simulink model "F16ASYM_Controlled_AoA"  (R2012b)
settings: Solver=ode3  SolverMode=SingleTasking  StartTime=0.0  StopTime=inf  FixedStep=T_sim  RelTol=1e-3
InitFcn:
  | load('NN_c_weights_Last_stable.mat')
values from neighbouring files (symbols this model uses):
  K_b_AoA = params(3)    [Cost_function.m]
  K_b_q = params(4)    [Cost_function.m]
  learning = 20    [Scheduling_desing.m]
  Model_used_flag = 1    [Scheduling_desing.m]
  reg_param = 0.5    [Scheduling_desing.m]
  T_sim = 0.02    [Scheduling_desing.m]
  tau_AoA = params(1)    [Cost_function.m]
  tau_q = params(2)    [Cost_function.m]
  Theta_1_roll_last = [0.00183613313267 0.00115998993235 0.0006676025148 0.00194921904952 0.00134963559861 0.00034352059664 0.000447169388141 0.00146749660935 0.00110199952389 7.77922383894e-05 0.00109492833348 0.00192687590535 ... (360 elements, 30x12)]    [NN_i_weights_LAST_STABLE.mat]
  Theta_2_roll_last = [0.000469743069697 0.000355923851088 0.00180035760697 0.00191855117771 0.00118851504447 0.0013331642065 0.0013164316578 0.000643981263341 0.00176817665434 0.000113802099363 0.000426534542462 0.00113815782354 ... (620 elements, 20x31)]    [NN_i_weights_LAST_STABLE.mat]
  Theta_3_roll_last = [9.62071520568e-05 -0.000389870886846 2.08260845013e-05 0.000140787743673 -0.000917525755397 -0.0014324207578 -0.00154701573815 -0.00131544476264 -0.00101205584381 5.06515794689e-05 -0.00111443483676 -0.00143957416141 ... (21 elements, 1x21)]    [NN_i_weights_LAST_STABLE.mat]
  V_long_lastA_w_z = [0.352826086601 -0.253633004548 -0.642535042878 0.237749930435 -0.618390629538 0.858074761295 0.268211230628 -0.448715080196 -0.0406384631192 0.401147605577 0.60598427709 0.0500551915851 ... (300 elements, 30x10)]    [NN_i_weights_LAST_STABLE.mat]
  V_long_lastAoA = [0.0774300162379 0.0911421319631 0.0352371192557 0.0542170286952 0.0651171200844 0.0177112012707 0.0982957728448 0.000259994642558 0.0194724569123 0.0466321328252 0.0556687953852 0.0252668067142 ... (300 elements, 30x10)]    [NN_i_weights_LAST_STABLE.mat]
  V_roll_last = [0.0540918675943 0.0557493347212 0.0839792276608 0.0460576391794 0.0671229058124 0.100220403067 0.0722493281881 0.0648875457457 0.00447599349201 0.0607299103823 0.0488037966361 0.0176785979393 ... (360 elements, 30x12)]    [NN_i_weights_LAST_STABLE.mat]
  V_yaw_last = [0.0965149149679 0.00833616709545 0.0365734360076 0.0523944217566 0.00790252078455 0.0700053845887 0.0345164868709 0.0111568465295 0.094060639546 0.0205483560006 0.000798047494256 0.0862769385758 ... (360 elements, 30x12)]    [NN_i_weights_LAST_STABLE.mat]
  velocity = M_eval_sche(I,J)*a    [Scheduling_desing.m]
  W_long_lastA_w_z = [-0.0522913429974 0.00385484301394 -0.00465489482472 -0.0139416219936 0.00295196421483 -0.013027768541 0.00585545058915 0.00278802233571 -0.00906272782329 -0.000396112031465 0.00405849743321 0.00509668457818 ... (31 elements, 1x31)]    [NN_i_weights_LAST_STABLE.mat]
  W_long_lastAoA = [-0.0192589013922 0.00873109909713 0.00432649597332 0.0420946902441 0.0293366820194 0.0351497798191 0.0234952374236 0.0360841187718 0.0112233388211 0.030147202199 0.0369533138617 0.00218839076415 ... (31 elements, 1x31)]    [NN_i_weights_LAST_STABLE.mat]
  W_roll_last = [-0.0006515532842 0.000535485585715 0.000550946920743 0.000806030945453 0.00045976209382 0.00065557954304 0.000945902185602 0.00070191398535 0.000635215543728 4.66501377412e-05 0.000597079583757 0.000485790566765 ... (31 elements, 1x31)]    [NN_i_weights_LAST_STABLE.mat]
  W_yaw_last = [-4.34263633305e-05 8.83823048922e-05 1.65575463724e-05 3.60293102233e-05 5.19752447623e-05 7.06399280852e-06 7.02425975821e-05 3.62680255076e-05 1.29996379937e-05 8.05072914397e-05 2.39941870661e-05 2.52427840574e-06 ... (31 elements, 1x31)]    [NN_i_weights_LAST_STABLE.mat]
undefined symbols (not defined in the file or in its folder): a1, alpha_map_eval, B, beta_map_eval, C_L_0, DiscIntNeverNeededParam, fi_flag_Simulink, G_eval, H_sq, H_sq_autotrim, k_B, m_B, M_sq, M_sq_autotrim, sigbuilder_block, Stall_curve, trim_control, trim_state, trim_throttle, V_Comp_A_w_z_last, V_Comp_last, V_roll_lastMOD, W_Comp_A_w_z_last, W_Comp_last, W_roll_lastMOD
libraries: Adaptive_FaultTolerantControl x43, dspsigops x29, F16_Actuator_Library x14, simulink x8, aerolibatmos2 x7, dsparch4 x6, simulink_extras x5, aerolibtransform2 x5, qcatlib x4, dspmtrx3 x3, dspvision x2, dspsnks4 x2
(part 1 of 11)
settings Model: MAModelExclusionFile=C:\Users\David\Documents\Estudios y formación academica\Cranfield\Thesis F16\Work\Solutions\7dof Base\F16ASYM_Controlled_exclusions.xml  Creator=David  LastModifiedBy=David
settings SolverCC: AutoInsertRateTranBlk=on
settings DataIOCC: SaveOutput=off  SignalLogging=off  DSMLogging=off  SaveTime=off
settings OptimizationCC: BlockReduction=off  InlineParams=on  InlineInvariantSignals=on  EnableMemcpy=off  StateBitsets=on  DataBitsets=on  UseTempVars=on  ZeroExternalMemoryAtStartup=off  ZeroInternalMemoryAtStartup=off  NoFixptDivByZeroProtection=on  EfficientMapNaN2IntZero=off  OptimizeModelRefInitCode=on  LifeSpan=1
settings HardwareCC: ProdIntDivRoundTo=Floor  ProdEndianess=LittleEndian  ProdHWDeviceType=Generic->Custom
settings RTWCC: SystemTargetFile=ert.tlc  TLCOptions=-p0  GenCodeOnly=on  TemplateMakefile=ert_default_tmf  Description=Embedded Coder  GenerateReport=on  RTWVerbose=off  ProcessScript=ert_make_rtw_hook  IncludeHyperlinkInReport=on  LaunchReport=on
settings CodeAppCC: ForceParamTrailComments=on  IgnoreCustomStorageClasses=off  SimulinkDataObjDesc=on  CustomSymbolStrGlobalVar=rt$N$M  CustomSymbolStrType=$N$M  CustomSymbolStrFcn=$N$M$F  CustomSymbolStrMacro=$N$M  InsertBlockDesc=on
settings ERTTargetCC: CodeReplacementLibrary=ISO_C  MultiwordLength=2048  GenerateSampleERTMain=on  IncludeMdlTerminateFcn=off  SuppressErrorStatus=on  SupportAbsoluteTime=off  SupportNonFinite=off  SupportComplex=off  PurelyIntegerCode=on  InlinedParameterPlacement=NonHierarchical  RootIOFormat=Structure reference  ERTCustomFileTemplate=example_file_process.tlc  ConvertIfToSwitch=off  SuppressUnreachableDefaultCases=off

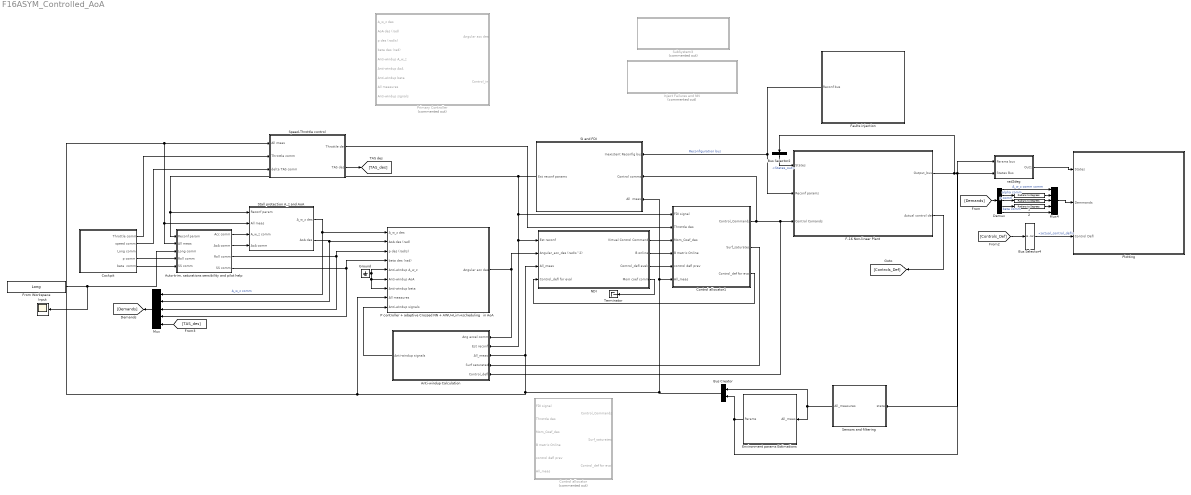
== system F16ASYM_Controlled_AoA ==
  "  " : simulink_extras/Transformations/Radians to Degrees
  "  1" : simulink_extras/Transformations/Radians to Degrees
  "  2" : simulink_extras/Transformations/Radians to Degrees
  Anti-windup Calculation : Subsystem  Variant=on  OverrideUsingVariant=Reconfigurable
  "Auto-trim, saturations sensibility and pilot help" : Subsystem
  Bus Creator : BusCreator  Inputs=2
  Bus Selector2 : BusSelector  OutputSignals=States_out
  Bus Selector4 : BusSelector  OutputSignals=actual_control_defl
  Cockpit : Subsystem
      mask Display:
      | image(imread('Cockpit2.jpg'))
      | 
      | port_label('output', 1, 'Throttle comm')
      | port_label('output', 2, 'Speed comm')
      | port_label('output', 3, 'Long comm')
      | port_label('output', 4, 'p comm')
      | port_label('output', 5, 'beta comm')
  Control allocator : Subsystem  Commented=on  Variant=on  OverrideUsingVariant=Control Allocator: NO RECONFIG
  Control allocator1 : Subsystem  Variant=on  OverrideUsingVariant=Control Allocator: RECONFIG
  Demux : Demux  Outputs=5
  Environment params Estimations : Subsystem
  F-16 Non-linear Plant : Subsystem  Variant=on  OverrideUsingVariant=Reconfigurable
      mask Display:
      | image(imread('f16.jpg'))
      | 
      | port_label('output', 1, 'Out_bus')
      | port_label('output', 2, 'Actual Control deflec')
      | 
      | port_label('input', 1, 'State_feedback')
      | port_label('input', 2, 'Reconf_params')
      | port_label('input', 3, 'Control_Commands')
      | 
      | % Variant dealing
      | ActiveVar = get_param(gcb,'activevariant');
      | 
      | 
      | disp(['{\bf\fontsize{16}',ActiveVar,'}'], 'texmode','on');
  Faults injection : Subsystem
      settings: OpenFcn=Control_GUI
      mask Display: disp(['{\bf \fontsize{16}',sprintf('Faults \n and\n  deviations\n  injection'),'}'], 'texmode','on');
  From Workspace : FromWorkspace  VariableName=Long  SampleTime=T_sim
  Ground : Ground
  Inject Failures and NN : Subsystem  Commented=on
      settings: OpenFcn=Control_GUI
      mask Display: disp('Inject Failures & NN management GUI')
  Input : Scope
      settings: YMin=-20  YMax=35  SaveName=ScopeData29
  Mux : Mux  Inputs=[1 1 1 1 1]
  Mux4 : Mux  Inputs=5
  NDI : Subsystem  Variant=on  OverrideUsingVariant=NDI: RECONFIG
  P controller + adaptive Crossed NN + AWU+Lim+scheduling   in AoA : Subsystem  VariantObject=Adaptive Controller Crossed+AWU+Lim
  Plotting : Subsystem
      mask Display:
      | disp('{\bf\fontsize{20} Plotting}', 'texmode','on');
      | % port_label('input', 1, 'States')
      | % port_label('input', 2, 'Demans')
  Primary Controller : Subsystem  Commented=on  Variant=on  OverrideUsingVariant=Adaptive Controller Crossed+AWU+Lim+hand-over
  SI and FDI : Subsystem  Variant=on  OverrideUsingVariant=Realistic
      mask Display:
      | % Variant dealing
      | ActiveVar = get_param(gcb,'activevariant');
      | 
      | 
      | 
      | disp(['{\bf \fontsize{14}',sprintf('SI \n&\nFDI\n\n '),ActiveVar,'}'], 'texmode','on');
  Sensors and filtering : Subsystem
  Speed-Throttle control : Subsystem
  Stall protection A_z and AoA : Subsystem  Variant=on  OverrideUsingVariant=Using AoA
  SubSystem3 : Subsystem  Commented=on
      settings: OpenFcn=FE_plot
      mask Display:
      | % image(imread('FE.png'))
      | 
      | disp('Flight Envelope position');
  Terminator : Terminator
  rad2deg : Subsystem
  wires:
  Sensors and filtering/1(All_measures) -> Environment params Estimations/1(All_meas), Bus Creator/1
  Control allocator1/2(Surf_saturated) -> Anti-windup Calculation/4(Surf saturated)
  NDI/1(Virtual Control Commands) -> Control allocator1/3(Mom_Coef_des)
  Ground/1 -> P controller + adaptive Crossed NN + AWU+Lim+scheduling   in AoA/7(Anti-windup beta), P controller + adaptive Crossed NN + AWU+Lim+scheduling   in AoA/6(Anti-windup AoA), P controller + adaptive Crossed NN + AWU+Lim+scheduling   in AoA/5(Anti-windup A_w_z)
  Bus Selector2/1 -> F-16 Non-linear Plant/1(States)  "<States_out>"
  NDI/2(B online) -> Control allocator1/4(B matrix Online)
  F-16 Non-linear Plant/2(Actual control def) -> [Controls_Def]
  P controller + adaptive Crossed NN + AWU+Lim+scheduling   in AoA/1(Angular acc des) -> NDI/2(Angular_acc_des (rad/s^2)), Anti-windup Calculation/1(Ang accel comm)
  NDI/3(Control_defl evald) -> Control allocator1/5(control defl prev)
  Control allocator1/3(Control_def for eval) -> NDI/4(Control_defl for eval)
  Faults injection/1(Reconf bus) -> F-16 Non-linear Plant/2(Reconf params), SI and FDI/1(Inexistent Reconfig bus)  "Reconfiguration bus"
  Control allocator1/1(Control_Commands) -> SI and FDI/2(Control comms), F-16 Non-linear Plant/3(Control Comands), Anti-windup Calculation/5(Control_defl)
  Bus Creator/1 -> Control allocator1/6(All_meas), SI and FDI/3(All  meas), P controller + adaptive Crossed NN + AWU+Lim+scheduling   in AoA/8(All measures), "Auto-trim, saturations sensibility and pilot help"/2(All meas), Stall protection A_z and AoA/2(All meas), Speed-Throttle control/1(All meas), NDI/3(All_meas), Anti-windup Calculation/3(All_meas)
  "Auto-trim, saturations sensibility and pilot help"/1(Acc comm) -> Stall protection A_z and AoA/3(A_w_z comm)
  Anti-windup Calculation/1(Anti-windup signals) -> P controller + adaptive Crossed NN + AWU+Lim+scheduling   in AoA/9(Anti-windup signals)
  Stall protection A_z and AoA/1(A_w_z des) -> Mux/1, P controller + adaptive Crossed NN + AWU+Lim+scheduling   in AoA/1(A_w_z des)  "A_w_z comm"
  "Auto-trim, saturations sensibility and pilot help"/4("SS comm ") -> P controller + adaptive Crossed NN + AWU+Lim+scheduling   in AoA/4(beta des (rad)), Mux/4
  "Auto-trim, saturations sensibility and pilot help"/3("Roll comm ") -> P controller + adaptive Crossed NN + AWU+Lim+scheduling   in AoA/3(p des (rad/s)), Mux/3
  SI and FDI/1(Est reconf params) -> "Auto-trim, saturations sensibility and pilot help"/1(Reconf param), Stall protection A_z and AoA/1(Reconf param), Control allocator1/1(FDI signal), Anti-windup Calculation/2(Est reconf), NDI/1(Est reconf)
  Cockpit/4(p comm) -> "Auto-trim, saturations sensibility and pilot help"/4(Roll comm)
  Cockpit/5(beta  comm) -> "Auto-trim, saturations sensibility and pilot help"/5(SS comm)
  "Auto-trim, saturations sensibility and pilot help"/2(AoA comm) -> Stall protection A_z and AoA/4(AoA comm)
  Cockpit/1(Throttle comm) -> Speed-Throttle control/2(Throttle comm)
  Cockpit/2(speed comm) -> Speed-Throttle control/3(delta TAS comm)
  Speed-Throttle control/1(Throttle des) -> Control allocator1/2(Throttle des)
  Mux/1 -> [Demands]
  Speed-Throttle control/2(TAS des) -> [TAS_des]
  [TAS_des] -> Mux/5
  Stall protection A_z and AoA/2(AoA des) -> Mux/2, P controller + adaptive Crossed NN + AWU+Lim+scheduling   in AoA/2(AoA des (rad))
  From Workspace/1 -> "Auto-trim, saturations sensibility and pilot help"/3(Long comm), Input/1
  NDI/4(Mom coef comm) -> Terminator/1
  rad2deg/1(Out1) -> Plotting/1(States)
  F-16 Non-linear Plant/1(Output_bus) -> rad2deg/2(States Bus), Sensors and filtering/1(state), Bus Selector2/1
  [Demands] -> Demux/1
  Environment params Estimations/1(Params) -> Bus Creator/2, rad2deg/1(Params bus)
  Demux/3 -> "  1"/1  "p comm"
  Demux/4 -> "  2"/1  "beta comm"
  Demux/2 -> "  "/1  "alpha comm"
  Mux4/1 -> Plotting/2(Demmands)
  Demux/1 -> Mux4/1  "A_w_z comm comm"
  "  "/1 -> Mux4/2
  "  1"/1 -> Mux4/3
  "  2"/1 -> Mux4/4
  [Controls_Def] -> Bus Selector4/1
  Bus Selector4/1 -> Plotting/3(Control Defl)  "<actual_control_defl>"
  Demux/5 -> Mux4/5

== system F16ASYM_Controlled_AoA/Anti-windup Calculation ==
  Ang accel comm : Inport
  Est reconf : Inport  Port=2
  All_meas : Inport  Port=3
  Surf saturated : Inport  Port=4
  Control_defl : Inport  Port=5
  Anti-windup: NO reconfigurable : Subsystem  VariantObject=No reconfigurable
  Anti-windup: Reconfigurable : Subsystem  VariantObject=Reconfigurable
  Anti-windup signals : Outport

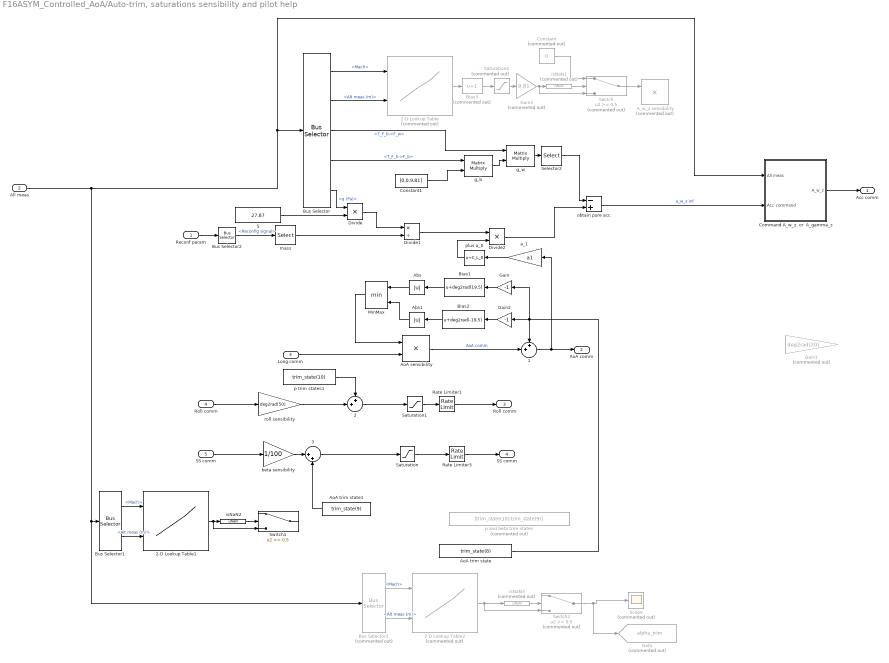
== system F16ASYM_Controlled_AoA/Auto-trim, saturations sensibility and pilot help ==
  Reconf param : Inport
  All meas : Inport  Port=2
  Long comm : Inport  Port=3
  Roll comm : Inport  Port=4
  SS comm : Inport  Port=5
  " 1" : Sum  Inputs=++|
  " 2" : Sum  Inputs=++|
  " 3" : Sum  Inputs=|++
  2-D Lookup Table : Lookup_n-D  Commented=on  BreakpointsForDimension1=M_sq  BreakpointsForDimension2=H_sq  Table=G_eval  RemoveProtectionInput=on  SampleTime=5*T_sim  RndMeth=Simplest  InputSameDT=on
  2-D Lookup Table1 : Lookup_n-D  BreakpointsForDimension1=M_sq_autotrim  BreakpointsForDimension2=H_sq_autotrim  Table=beta_map_eval  RemoveProtectionInput=on  SampleTime=5*T_sim  RndMeth=Simplest  InputSameDT=on
  2-D Lookup Table2 : Lookup_n-D  Commented=on  BreakpointsForDimension1=M_sq_autotrim  BreakpointsForDimension2=H_sq_autotrim  Table=alpha_map_eval  RemoveProtectionInput=on  SampleTime=5*T_sim  RndMeth=Simplest  InputSameDT=on
  A_w_z sensibility : Product  Commented=on  Inputs=**
  Abs : Abs
  Abs1 : Abs
  AoA sensibility : Product  Inputs=**
  AoA trim state : Constant  Value=trim_state(8)
  AoA trim state1 : Constant  Value=trim_state(9)
  Bias1 : Bias  Bias=deg2rad(19.5)
  Bias2 : Bias  Bias=deg2rad(-19.5)
  Bias3 : Bias  Commented=on  Bias=1
  Bus Selector : BusSelector  OutputSignals=signal2.Mach,signal1.Alt meas (m),signal2.T_F_b->F_w,signal2.T_F_h->F_b,signal2.q (Pa)
  Bus Selector1 : BusSelector  OutputSignals=signal2.Mach,signal1.Alt meas (m)
  Bus Selector2 : BusSelector  OutputSignals=Reconfig signal
  Bus Selector3 : BusSelector  Commented=on  OutputSignals=signal2.Mach,signal1.Alt meas (m)
  Command A_w_z  or  A_gamma_z : Subsystem  mask{Crit=A_w_z, Criteria=0}
      mask prompts: Crit "Commdn in:"
      mask init:
      | val = get_param(gcb,'MaskValues');
      | switch lower(val{1})
      |  case 'A_w_z'
      |      Criteria=0;
      |  case 'A_gamma_z'
      |      Criteria=1;
      | end
      mask TypeOptions Crit: A_w_z | A_gamma_z
      mask Display:
      | val = get_param(gcb,'MaskValues');
      | 
      | disp(['{\bf\fontsize{16}',upper(val{1}),'}'], 'texmode','on');
  Constant : Constant  Commented=on  Value=0
  Constant1 : Constant  Value=[0,0,9.81]
  Divide : Product  Inputs=**
  Divide1 : Product  Inputs=*/
  Divide2 : Product  Inputs=**
  Gain : Gain  Gain=-1
  Gain1 : Gain  Commented=on  Gain=deg2rad(20)
  Gain2 : Gain  Gain=-1
  Gain3 : Gain  Commented=on  Gain=9.81
  Goto : Goto  Commented=on  GotoTag=alpha_trim  TagVisibility=global
  MinMax : MinMax  Inputs=2
  Rate Limiter1 : RateLimiter  RisingSlewLimit=deg2rad(100)  FallingSlewLimit=-deg2rad(100)  SampleTimeMode=inherited  InitialCondition=trim_state(10)
  Rate Limiter3 : RateLimiter  RisingSlewLimit=deg2rad(8)  FallingSlewLimit=-deg2rad(8)  SampleTimeMode=inherited  InitialCondition=trim_state(9)
  S : Constant  Value=27.87
  Saturation : Saturate  UpperLimit=deg2rad(15)  LowerLimit=deg2rad(-15)
  Saturation1 : Saturate  UpperLimit=deg2rad(50)  LowerLimit=deg2rad(-50)
  Saturation2 : Saturate  Commented=on  UpperLimit=9  LowerLimit=0
  Scope : Scope  Commented=on
      settings: YMin=0  YMax=0.175  SaveName=ScopeData26
  Selector2 : Selector  InputPortWidth=3  IndexOptions=Index vector (dialog)  Indices=3  OutputSizes=1
  Switch : Switch  Commented=on  Threshold=0.5
  Switch1 : Switch  Threshold=0.5
  Switch2 : Switch  Commented=on  Threshold=0.5
  a_1 : Gain  Gain=a1
  beta sensibility : Gain  Gain=1/100
  g_b : Product  Multiplication=Matrix(*)
  g_w : Product  Multiplication=Matrix(*)
  isNaN1 : RelationalOperator  Commented=on  Operator=isNaN  OutDataTypeStr=boolean
  isNaN2 : RelationalOperator  Operator=isNaN  OutDataTypeStr=boolean
  isNaN3 : RelationalOperator  Commented=on  Operator=isNaN  OutDataTypeStr=boolean
  mass : Selector  InputPortWidth=19  IndexOptions=Index vector (dialog)  Indices=1  OutputSizes=1
  obtain pure acc : Sum  Inputs=-+
  p and beta trim states : Constant  Commented=on  Value=[trim_state(10);trim_state(9)]
  p trim states1 : Constant  Value=trim_state(10)
  plus a_0 : Bias  Bias=C_L_0
  roll sensibility : Gain  Gain=deg2rad(50)
  Acc comm : Outport
  AoA comm : Outport  Port=2
  "Roll comm " : Outport  Port=3
  "SS comm " : Outport  Port=4
  wires:
  SS comm/1 -> beta sensibility/1
  Roll comm/1 -> roll sensibility/1
  Rate Limiter3/1 -> "SS comm "/1
  Rate Limiter1/1 -> "Roll comm "/1
  Saturation/1 -> Rate Limiter3/1
  Saturation1/1 -> Rate Limiter1/1
  Command A_w_z  or  A_gamma_z/1(A_w_z) -> Acc comm/1
  Reconf param/1 -> Bus Selector2/1
  " 1"/1 -> a_1/1, AoA comm/1
  Switch2/1 -> Goto/1, Scope/1
  Bus Selector/1 -> 2-D Lookup Table/1  "<Mach>"
  Bus Selector/2 -> 2-D Lookup Table/2  "<Alt meas (m)>"
  2-D Lookup Table/1 -> Bias3/1
  Switch/1 -> A_w_z sensibility/1
  Long comm/1 -> AoA sensibility/2
  " 3"/1 -> Saturation/1
  " 2"/1 -> Saturation1/1
  AoA sensibility/1 -> " 1"/2  "AoA comm"
  Gain/1 -> Bias1/1
  Gain2/1 -> Bias2/1
  Bias1/1 -> Abs/1
  Bias2/1 -> Abs1/1
  MinMax/1 -> AoA sensibility/1
  Abs/1 -> MinMax/1
  Abs1/1 -> MinMax/2
  Constant/1 -> Switch/1
  isNaN1/1 -> Switch/2
  Gain3/1 -> isNaN1/1, Switch/3
  Saturation2/1 -> Gain3/1
  Bias3/1 -> Saturation2/1
  p trim states1/1 -> " 2"/1
  All meas/1 -> Command A_w_z  or  A_gamma_z/1(All meas), Bus Selector/1, Bus Selector1/1, Bus Selector3/1
  Bus Selector1/1 -> 2-D Lookup Table1/1  "<Mach>"
  Bus Selector1/2 -> 2-D Lookup Table1/2  "<Alt meas (m)>"
  Bus Selector3/2 -> 2-D Lookup Table2/2  "<Alt meas (m)>"
  Bus Selector3/1 -> 2-D Lookup Table2/1  "<Mach>"
  isNaN2/1 -> Switch1/2
  2-D Lookup Table1/1 -> Switch1/3, isNaN2/1
  isNaN3/1 -> Switch2/2
  2-D Lookup Table2/1 -> Switch2/3, isNaN3/1
  beta sensibility/1 -> " 3"/1
  roll sensibility/1 -> " 2"/2
  AoA trim state/1 -> " 1"/1, Gain/1, Gain2/1
  Bus Selector2/1 -> mass/1  "<Reconfig signal>"
  Divide/1 -> Divide1/1
  mass/1 -> Divide1/2
  S/1 -> Divide/2
  Bus Selector/5 -> Divide/1  "<q (Pa)>"
  a_1/1 -> plus a_0/1
  Divide1/1 -> Divide2/1
  plus a_0/1 -> Divide2/2
  Bus Selector/3 -> g_w/1  "<T_F_b->F_w>"
  Bus Selector/4 -> g_b/1  "<T_F_h->F_b>"
  Constant1/1 -> g_b/2
  g_b/1 -> g_w/2
  g_w/1 -> Selector2/1
  obtain pure acc/1 -> Command A_w_z  or  A_gamma_z/2(Acc command)  "a_w_z inf"
  Divide2/1 -> obtain pure acc/2
  Selector2/1 -> obtain pure acc/1
  AoA trim state1/1 -> " 3"/2

== system F16ASYM_Controlled_AoA/Cockpit ==
  Add : Sum  Commented=on  Inputs=++++
  Degrees to Radians : simulink_extras/Transformations/Degrees to Radians
  Delay : Delay  Commented=on  DelayLength=1300
  Demux2 : Demux  Outputs=3
  Joystick : Subsystem  Commented=on
  Manual Switch1 : ManualSwitch  CurrentSetting=0
  Mux1 : Mux  Inputs=3
  Mux2 : Mux  Commented=on  Inputs=3
  Signal Builder1 : Subsystem  Tag=STV Subsys  Commented=on  LoadFcn=sigbuilder_block('load');  StartFcn=sigbuilder_block('start');  StopFcn=sigbuilder_block('stop');  ClipboardFcn=sigbuilder_block('clipboard');  mask(Sigbuilder block){}
      mask help: Simulink:masks:SigbuilderBlock_MD
      mask init:
      | if ~strcmp(get_param(bdroot(gcbh),'SimulationStatus'),'stopped') tuvar = sigbuilder_block('maskInit'); end
      settings: CopyFcn=sigbuilder_block('copy');  DeleteFcn=sigbuilder_block('delete');  ModelCloseFcn=sigbuilder_block('modelClose');  PreSaveFcn=sigbuilder_block('preSave');  PauseFcn=sigbuilder_block('pause');  ContinueFcn=sigbuilder_block('continue');  NameChangeFcn=sigbuilder_block('namechange');  OpenFcn=sigbuilder_block('open',[6 28.5 1012.5 484.5 ]);  CloseFcn=sigbuilder_block('close');
      mask Display: plot(0, 0, 100, 100,[2, 2, 32, 32, 2], [68, 8, 8, 68, 68],[32, 2], [38, 38], [32, 19, 2],[53, 60, 44], [32, 17, 17, 2],[16, 16, 31, 31]);txt = getActiveGroup(gcbh);text(2, 100, txt,'verticalAlignment', 'top');
  Signal Builder2 : Subsystem  Tag=STV Subsys  Commented=on  LoadFcn=sigbuilder_block('load');  StartFcn=sigbuilder_block('start');  StopFcn=sigbuilder_block('stop');  ClipboardFcn=sigbuilder_block('clipboard');  mask(Sigbuilder block){}
      mask help: Simulink:masks:SigbuilderBlock_MD
      mask init:
      | if ~strcmp(get_param(bdroot(gcbh),'SimulationStatus'),'stopped') tuvar = sigbuilder_block('maskInit'); end
      settings: CopyFcn=sigbuilder_block('copy');  DeleteFcn=sigbuilder_block('delete');  ModelCloseFcn=sigbuilder_block('modelClose');  PreSaveFcn=sigbuilder_block('preSave');  PauseFcn=sigbuilder_block('pause');  ContinueFcn=sigbuilder_block('continue');  NameChangeFcn=sigbuilder_block('namechange');  OpenFcn=sigbuilder_block('open',[6 28.5 1012.5 484.5 ]);  CloseFcn=sigbuilder_block('close');
      mask Display: plot(0, 0, 100, 100,[2, 2, 32, 32, 2], [68, 8, 8, 68, 68],[32, 2], [38, 38], [32, 19, 2],[53, 60, 44], [32, 17, 17, 2],[16, 16, 31, 31]);txt = getActiveGroup(gcbh);text(2, 100, txt,'verticalAlignment', 'top');
  Throttle comm : Outport
  speed comm : Outport  Port=2
  Long comm : Outport  Port=3
  p comm : Outport  Port=4
  beta  comm : Outport  Port=5
  wires:
  Manual Switch1/1 -> Demux2/1
  Joystick/5(sideslip) -> Mux2/3
  Joystick/4(Roll) -> Mux2/2
  Joystick/2(Throttle) -> Throttle comm/1
  Mux2/1 -> Manual Switch1/1
  Joystick/3(Long: Acc) -> Mux2/1
  Demux2/1 -> Long comm/1
  Signal Builder1/1(Signal 1) -> Add/1
  Signal Builder1/2(Signal 5) -> Add/2
  Signal Builder1/4(Signal 7) -> Add/4
  Signal Builder1/3(Signal 6) -> Add/3
  Signal Builder2/2(Signal 2) -> Mux1/2
  Signal Builder2/4(Signal 4) -> Mux1/3
  Joystick/1(speed des) -> speed comm/1
  Add/1 -> Delay/1
  Demux2/2 -> p comm/1  "p comm"
  Demux2/3 -> beta  comm/1  "beta comm"
  Degrees to Radians/1 -> Manual Switch1/2
  Mux1/1 -> Degrees to Radians/1

== system F16ASYM_Controlled_AoA/Control allocator ==
  FDI signal : Inport
  Throttle des : Inport  Port=2
  Mom_Coef_des : Inport  Port=3
  B matrix Online : Inport  Port=4
  control defl prev : Inport  Port=5
  All_meas : Inport  Port=6
  Control allocator: NO RECONF : Subsystem  RTWFcnName=abc  RTWFileName=asas  VariantObject=Control Allocator: NO RECONFIG
      settings: MinAlgLoopOccurrences=on  RTWFcnNameOpts=User specified  RTWFileNameOpts=User specified
  Control allocator: RECONFIG : Subsystem  RTWFcnName=abc  RTWFileName=asas  VariantObject=Control Allocator: RECONFIG
      settings: MinAlgLoopOccurrences=on  RTWFcnNameOpts=User specified  RTWFileNameOpts=User specified
  Control_Commands : Outport
  Surf_saturated : Outport  Port=2
  Control_def for eval : Outport  Port=3

== system F16ASYM_Controlled_AoA/Control allocator1 ==
  FDI signal : Inport
  Throttle des : Inport  Port=2
  Mom_Coef_des : Inport  Port=3
  B matrix Online : Inport  Port=4
  control defl prev : Inport  Port=5
  All_meas : Inport  Port=6
  Control allocator: NO RECONF : Subsystem  RTWFcnName=abc  RTWFileName=asas  VariantObject=Control Allocator: NO RECONFIG
      settings: MinAlgLoopOccurrences=on  RTWFcnNameOpts=User specified  RTWFileNameOpts=User specified
  Control allocator: RECONFIG : Subsystem  RTWFcnName=abc  RTWFileName=asas  VariantObject=Control Allocator: RECONFIG
      settings: MinAlgLoopOccurrences=on  RTWFcnNameOpts=User specified  RTWFileNameOpts=User specified
  Control_Commands : Outport
  Surf_saturated : Outport  Port=2
  Control_def for eval : Outport  Port=3

== system F16ASYM_Controlled_AoA/Environment params Estimations ==
  note: Acceleration of the body in body axes
  note: Acceleration of the body
      |   in wind axes
  All_meas : Inport
  ALT_and_M_GAIN_LIST : Gain
  A_b_CG : Product  Multiplication=Matrix(*)
  A_w_CG : Product  Multiplication=Matrix(*)
  Bias : Bias  Bias=-[0;0;1]
  Bus Creator : BusCreator  Inputs=8
  Bus Selector : BusSelector  OutputSignals=V_TAS (m/s),Alt meas (m),AoA meas (rad),SS meas (rad),Euler meas (rad),an_b_CG meas
  Constant : Constant  Value=0
  Direction Cosine Matrix Body to Wind T_F_b->F_w : aerolibtransform2/Direction Cosine Matrix Body to Wind
  Divide : Product  Inputs=**
  Gain : Gain  Gain=1/2
  Gain1 : Gain  Gain=-1*9.81
  Gain2 : Gain  Gain=-1
  Gain3 : Gain  Gain=-1
  ISA Atmosphere Model : aerolibatmos2/ISA Atmosphere Model  custom=off  g=9.80665  gamma=1.4  R=287.0531  L=0.0065  h_trop=11000  h_strat=20000  rho0=1.225  P0=101325  T0=288.15
  Mach number : Subsystem
  Matrix Multiply1 : Product  Multiplication=Matrix(*)
  Mux : Mux  Inputs=2
  Mux1 : Mux  Inputs=3
  Mux2 : Mux  Inputs=2
  Rotation Angles to Direction Cosine Matrix: F_b->F_T : aerolibtransform2/Rotation Angles to Direction Cosine Matrix  rotationOrder=ZYX
  Rotation Angles to Direction Cosine Matrix: F_h->F_b : aerolibtransform2/Rotation Angles to Direction Cosine Matrix  rotationOrder=ZYX
  Selector1 : Selector  InputPortWidth=3  IndexOptions=Index vector (dialog)  Indices=[3 2 1]  OutputSizes=1
  Selector7 : Selector  InputPortWidth=3  IndexOptions=Index vector (dialog)  Indices=[3 2 1]  OutputSizes=1
  Terminator : Terminator
  Terminator1 : Terminator
  Terminator2 : Terminator
  Transpose : dspmtrx3/Transpose  Hermitian=off  overflowFlag=off
  dyn pressure : Product  Inputs=**
  Params : Outport
  wires:
  All_meas/1 -> Bus Selector/1
  Bus Selector/1 -> Mach number/1(V), Divide/1, Divide/2  "<V_TAS (m/s)>"
  Bus Selector/2 -> Mux2/1, ISA Atmosphere Model/1  "<Alt meas (m)>"
  ISA Atmosphere Model/4 -> dyn pressure/2
  dyn pressure/1 -> Bus Creator/1  "q (Pa)"
  Bus Creator/1 -> Params/1
  Divide/1 -> Gain/1
  Gain/1 -> dyn pressure/1
  Bus Selector/3 -> Mux/1, Gain2/1  "<AoA meas (rad)>"
  Bus Selector/4 -> Gain3/1, Mux/2  "<SS meas (rad)>"
  Mux/1 -> Direction Cosine Matrix Body to Wind T_F_b->F_w/1
  Bus Selector/6 -> Matrix Multiply1/2  "<an_b_CG meas >"
  Bus Selector/5 -> Selector7/1  "<Euler meas (rad)>"
  Selector7/1 -> Rotation Angles to Direction Cosine Matrix: F_h->F_b/1
  Rotation Angles to Direction Cosine Matrix: F_h->F_b/1 -> Transpose/1, Bus Creator/8, A_b_CG/1  "T_F_h->F_b"
  Matrix Multiply1/1 -> Bias/1
  Transpose/1 -> Matrix Multiply1/1
  Bias/1 -> Gain1/1
  A_b_CG/1 -> Bus Creator/7, A_w_CG/2  "A_b_CG"
  A_w_CG/1 -> Bus Creator/6  "A_w_CG"
  Gain1/1 -> A_b_CG/2
  Direction Cosine Matrix Body to Wind T_F_b->F_w/1 -> A_w_CG/1, Bus Creator/5  "T_F_b->F_w"
  Selector1/1 -> Rotation Angles to Direction Cosine Matrix: F_b->F_T/1
  Rotation Angles to Direction Cosine Matrix: F_b->F_T/1 -> Bus Creator/4  "T_F_b->F_T"
  Gain2/1 -> Mux1/1
  Gain3/1 -> Mux1/3
  Constant/1 -> Mux1/2
  Mux1/1 -> Selector1/1
  ISA Atmosphere Model/2 -> Bus Creator/3, Mach number/2(a)  "a"
  Mach number/1(Mach) -> Mux2/2, Bus Creator/2  "Mach"
  ISA Atmosphere Model/1 -> Terminator/1
  ISA Atmosphere Model/3 -> Terminator1/1  "Pressure (Pa)"
  Mux2/1 -> ALT_and_M_GAIN_LIST/1
  ALT_and_M_GAIN_LIST/1 -> Terminator2/1

== system F16ASYM_Controlled_AoA/F-16 Non-linear Plant ==
  States : Inport
  Reconf params : Inport  Port=2
  Control Comands : Inport  Port=3
  SYM and ASYM model: No reconfigurable : Subsystem  VariantObject=No Reconfigurable
  SYM and ASYM model: RECONFIGURABLE : Subsystem  VariantObject=Reconfigurable
  Output_bus : Outport
  Actual control def : Outport  Port=2

== system F16ASYM_Controlled_AoA/Faults injection ==
  note: Blockades now:
      | Input 1 to fixed controller at the current position
      | 0 otherwise
  note: Blockades: Input any number to fixed the
      | surface there. If non NaN
  note: RECONFIGURATION PARAMETERS
      |
      | 24. mass  Estimated mass
      | 25. S_current_L
      | 26. S_current_R
      | 27. S_fin_current
      | 28. x_cg
      | 29. Jy
      | 30. Jxz
      | 31. Jz
      | 32. Jx
      | 33. EFF_el_L
      | 34. EFF_el_R
      | 35. EFF_ail_L
      | 36. EFF_ail_R
      | 37. EFF_rud
      | 38. EFF_lef_L
      | 39. EFF_lef_R
      | 40. Delta_C_Lift_X
      | 41. Delta_C_Drag_X
      | 42. Delta_C_m_X
  Blockades at : Constant  Value="[NaN  NaN  NaN  NaN  NaN  NaN  NaN]"  SampleTime=T_sim
  Blockades now : Constant  Value="[0  0  0  0  0  0  0]"  SampleTime=T_sim
  Bus Creator : BusCreator  Inputs=3
  Delta_J : Constant  Value="[0  0  0  0]"  SampleTime=T_sim
  MATLAB Function : MATLAB Function  TreatAsAtomicUnit=on
  Transpose : dspmtrx3/Transpose  Hermitian=off  overflowFlag=off
  delta_S_L : Constant  Value=[0]  SampleTime=T_sim
  delta_S_R : Constant  Value=[0]  SampleTime=T_sim
  delta_S_fin : Constant  Value=[0]  SampleTime=T_sim
  delta_coef : Constant  Value="[0  0  0]"  SampleTime=T_sim
  delta_mass : Constant  Value=[0]  SampleTime=T_sim
  effectiveness : Constant  Value="[1  1  1  1  1  1  1]"  SampleTime=T_sim
  xcg : Constant  Value=[0.3]  SampleTime=T_sim
  Reconf bus : Outport
  wires:
  MATLAB Function/1(reconfig_params) -> Bus Creator/1  "Reconfig signal"
  Bus Creator/1 -> Reconf bus/1
  Blockades at/1 -> Bus Creator/2  "Blockades"
  Blockades now/1 -> Transpose/1
  Transpose/1 -> Bus Creator/3  "Blockade now"
  delta_mass/1 -> MATLAB Function/1(Delta_mass)
  delta_S_L/1 -> MATLAB Function/2(Delta_S_L)
  delta_S_R/1 -> MATLAB Function/3(Delta_S_R)
  delta_S_fin/1 -> MATLAB Function/4(Delta_S_Fin)
  xcg/1 -> MATLAB Function/5(xcg)
  Delta_J/1 -> MATLAB Function/6(Delta_J)
  effectiveness/1 -> MATLAB Function/7(Eff)
  delta_coef/1 -> MATLAB Function/8(Deltas_coef)

== system F16ASYM_Controlled_AoA/Inject Failures and NN ==

== system F16ASYM_Controlled_AoA/NDI ==
  Est reconf : Inport
  Angular_acc_des (rad/s^2) : Inport  Port=2
  All_meas : Inport  Port=3
  Control_defl for eval : Inport  Port=4
  NDI: NO RECONFIG : Subsystem  RTWFcnName=abc  RTWFileName=asas  VariantObject=NDI: NO RECONFIG
      settings: RTWFcnNameOpts=User specified  RTWFileNameOpts=User specified
  NDI: RECONFIG : Subsystem  RTWFcnName=abc  RTWFileName=asas  VariantObject=NDI: RECONFIG
      settings: RTWFcnNameOpts=User specified  RTWFileNameOpts=User specified
  Virtual Control Commands : Outport
  B online : Outport  Port=2
  Control_defl evald : Outport  Port=3
  Mom coef comm : Outport  Port=4

== system F16ASYM_Controlled_AoA/P controller + adaptive Crossed NN + AWU+Lim+scheduling   in AoA ==
  A_w_z des : Inport
  AoA des (rad) : Inport  Port=2
  p des (rad/s) : Inport  Port=3
  beta des (rad) : Inport  Port=4
  Anti-windup A_w_z : Inport  Port=5
  Anti-windup AoA : Inport  Port=6
  Anti-windup beta : Inport  Port=7
  All measures : Inport  Port=8
  Anti-windup signals : Inport  Port=9
  Body Rates Controller : Subsystem
  Bus Creator : BusCreator  Inputs=3
  Bus Creator1 : BusCreator  Inputs=2
  Bus Creator2 : BusCreator
  Bus Creator3 : BusCreator  Inputs=2
  Bus Selector3 : BusSelector  OutputSignals=signal1.SS meas (rad)
  Complete crossed On-line (adaptive) multi-layer NN: AoA : Subsystem  VariantObject=NN on AoA
  Display{,1..3,5..6} (6 alike) : Display
  "Display4 " : Display
  Lat_dir Dyn Inversion: beta_dot->r_c : Subsystem
  Long Dyn Inversion: alpha_dot ->q : Subsystem
  Longitudinal controller in AoA : Subsystem  VariantObject=Controller of AoA
  Memory : Memory  X0=[0,0,0]
  Physical limitation : Subsystem
  Ref Model and P Controller : Adaptive_FaultTolerantControl/Ref Model and P Controller  tau=0.45  y_i=trim_state(9)  K_f=1  K_b=5
  Scope1 : Scope
      settings: YMin=-8000  YMax=9000  SaveName=ScopeData27
  "Sigmoid " : Subsystem  mask{a=0.15}
      mask prompts: a "Sigmoid a param"
      mask TypeOptions a: a/Value
      mask Display:
      | x=-25:0.1:25;
      | 
      | y=(2.0 ./ (1.0 + exp(-a.*x))-1) ;
      | y2=zeros(size(x));
      | 
      | plot(x,y,x,y2);
      | 
      | text(-12,0.5, ['a= ',num2str(a)])
  Sum : Sum  Inputs=-+|
  Sum1 : Sum  Inputs=+-|
  Terminator1 : Terminator
  Angular acc des : Outport
  wires:
  Lat_dir Dyn Inversion: beta_dot->r_c/1(r_c) -> Display6/1, Body Rates Controller/3(r_ref)
  Bus Selector3/1 -> Ref Model and P Controller/2  "<SS meas (rad)>"
  p des (rad/s)/1 -> Body Rates Controller/1(p_ref)
  Long Dyn Inversion: alpha_dot ->q/1(q_c) -> Body Rates Controller/2(q_ref), Display1/1
  beta des (rad)/1 -> Ref Model and P Controller/1
  Longitudinal controller in AoA/2(alpha_dot_c) -> Long Dyn Inversion: alpha_dot ->q/1(alpha_dot_c), Display/1
  AoA des (rad)/1 -> Longitudinal controller in AoA/2(AoA des (rad))
  Anti-windup AoA/1 -> Longitudinal controller in AoA/4(Anti-windup AoA)
  Anti-windup A_w_z/1 -> Longitudinal controller in AoA/3(Anti-windup A_w_z)
  A_w_z des/1 -> Longitudinal controller in AoA/1(A_w_z des)
  Sum/1 -> "Display4 "/1, "Sigmoid "/1(In), Physical limitation/1(v comm)  "v"
  All measures/1 -> Complete crossed On-line (adaptive) multi-layer NN: AoA/2(All_meas), Longitudinal controller in AoA/5(All meas), Physical limitation/2(all meas), Body Rates Controller/4(All_meas), Lat_dir Dyn Inversion: beta_dot->r_c/2(All_meas), Bus Selector3/1, Long Dyn Inversion: alpha_dot ->q/2(All_meas)
  Body Rates Controller/4(Angular acc des (rad/s^2)) -> Display3/1, Sum/2  "v_p+v_dot_ff"
  Bus Creator/1 -> Complete crossed On-line (adaptive) multi-layer NN: AoA/3(NN variables)
  Memory/1 -> Complete crossed On-line (adaptive) multi-layer NN: AoA/1(v_ad^ prev)
  Body Rates Controller/2(p_chanel vars) -> Bus Creator/2  "p_chanel_vars"
  Body Rates Controller/1(q_chanel vars) -> Bus Creator1/2  "q_chanel_vars"
  Longitudinal controller in AoA/1(alpha_chanel vars) -> Bus Creator1/1  "alpha_chanel vars"
  Bus Creator1/1 -> Bus Creator/1  "Long chanel"
  Ref Model and P Controller/2 -> Bus Creator2/1  "beta_sf_dot"
  Ref Model and P Controller/3 -> Sum1/1, Bus Creator2/2  "beta_sf"
  Sum1/1 -> Bus Creator2/3  "beta_err"
  Ref Model and P Controller/4 -> Sum1/2
  Ref Model and P Controller/5 -> Bus Creator2/4  "K_b_beta"
  Body Rates Controller/3(r_chanel vars) -> Bus Creator3/1  "r_chanel vars"
  Bus Creator2/1 -> Bus Creator3/2  "beta_chanel vars"
  Bus Creator3/1 -> Bus Creator/3  "beta_r_chanel"
  Anti-windup beta/1 -> Terminator1/1
  "Sigmoid "/1(Out) -> Memory/1
  Complete crossed On-line (adaptive) multi-layer NN: AoA/1(v_ad^) -> Scope1/1, Display2/1, Sum/1  "v_ad^"
  Ref Model and P Controller/1 -> Display5/1, Lat_dir Dyn Inversion: beta_dot->r_c/1(beta_dot_c)
  Physical limitation/1(v limted) -> Angular acc des/1
  Anti-windup signals/1 -> Complete crossed On-line (adaptive) multi-layer NN: AoA/4(AWU)

== system F16ASYM_Controlled_AoA/Plotting ==
  States : Inport
  Demmands : Inport  Port=2
  Control Defl : Inport  Port=3
  Demux : Demux  Outputs=5
  Demux1 : Demux  Outputs=20
  Mux1 : Mux  Inputs=2
  Mux4 : Mux  Inputs=2
  Performance : ToWorkspace  VariableName=PERFORMANCE_AoA  SampleTime=-1  SaveFormat=Timeseries
  Terminator{,1..22} (23 alike) : Terminator
  wires:
  Demux1/8 -> Mux1/2  "alpha( deg)"
  States/1 -> Demux1/1
  Demmands/1 -> Demux/1
  Mux1/1 -> Performance/1
  Demux/2 -> Mux1/1  "alpha comm"
  Demux/1 -> Mux4/1  "A_w_z comm"
  Demux1/1 -> Terminator/1  "npos   (m)"
  Demux1/2 -> Terminator1/1  "epos   (m)"
  Demux1/3 -> Terminator2/1  "alt   (m)"
  Demux1/4 -> Terminator3/1  "phi   (deg)"
  Demux1/5 -> Terminator4/1  "theta   (deg)"
  Demux1/6 -> Terminator5/1  "psi  (deg)"
  Demux1/7 -> Terminator8/1  "TAS   (m/s)"
  Demux1/9 -> Terminator6/1  "beta  (deg)"
  Demux1/10 -> Terminator7/1  "p   (deg/s)"
  Demux1/11 -> Terminator9/1  "q   (deg/s)"
  Demux1/12 -> Terminator10/1  "r   (deg/s)"
  Demux1/13 -> Terminator11/1  "pow"
  Demux1/14 -> Terminator12/1  "nx (g)"
  Demux1/15 -> Terminator13/1  "ny (g)"
  Demux1/16 -> Terminator14/1  "nz (g)"
  Demux1/17 -> Terminator15/1  "mach"
  Demux1/18 -> Terminator16/1  "qbar (Pa"
  Demux1/19 -> Terminator17/1  "ps (Pa)"
  Demux1/20 -> Mux4/2  "A_w_z"
  Demux/3 -> Terminator19/1  "p comm"
  Demux/4 -> Terminator20/1  "beta comm"
  Demux/5 -> Terminator21/1  "TAS comm"
  Control Defl/1 -> Terminator22/1
  Mux4/1 -> Terminator18/1

== system F16ASYM_Controlled_AoA/Primary Controller ==
  A_w_z des : Inport
  AoA des (rad) : Inport  Port=2
  p des (rad/s) : Inport  Port=3
  beta des (rad) : Inport  Port=4
  Anti-windup A_w_z : Inport  Port=5
  Anti-windup AoA : Inport  Port=6
  Anti-windup beta : Inport  Port=7
  All measures : Inport  Port=8
  Anti-windup signals : Inport  Port=9
  P  + Crossed NN + AWU+Lim + hand-over : Subsystem  VariantObject=Adaptive Controller Crossed+AWU+Lim+hand-over
  P controller : Subsystem  VariantObject=P Controller
  P controller + adaptive Crossed NN : Subsystem  VariantObject=Adaptive Controller Crossed
  "P controller + adaptive Crossed NN + AWU+Lim " : Subsystem  VariantObject=Adaptive Controller Crossed+AWU+Lim
  P controller + adaptive Isolated NN : Subsystem  VariantObject=Adaptive Controller Isolated
  PI Primary Controller : Subsystem  VariantObject=PI Controller
  Angular acc des : Outport
  Control_in : Outport  Port=2

== system F16ASYM_Controlled_AoA/SI and FDI ==
  Inexistent Reconfig bus : Inport
  Control comms : Inport  Port=2
  All  meas : Inport  Port=3
  SI and FDI: Realistic : Subsystem  VariantObject=Realistic
  SI and FDI: Unrealistic : Subsystem  VariantObject=Unrealistic
  Est reconf params : Outport

== system F16ASYM_Controlled_AoA/Sensors and filtering ==
  note: This is measured load factor
  note: Add noise, uncertainty and delay here!!!
  state : Inport
  Bus Creator : BusCreator  Inputs=8
  Bus Selector2 : BusSelector  OutputSignals=X_e,TAS,alpha ; beta,p;q;r,euler,an_b_CG,Throttle
  Demux : Demux  Outputs=3
  Demux1 : Demux  Outputs=2
  Gain{,1..4} (5 alike) : Gain
  Terminator : Terminator
  Terminator1 : Terminator
  All_measures : Outport
  wires:
  state/1 -> Bus Selector2/1
  Bus Selector2/1 -> Demux/1  "<X_e>"
  Demux/3 -> Bus Creator/1  "Alt meas (m)"
  Demux/1 -> Terminator/1
  Demux/2 -> Terminator1/1
  Bus Selector2/2 -> Gain/1  "<TAS>"
  Bus Selector2/3 -> Demux1/1  "<alpha ; beta>"
  Demux1/1 -> Bus Creator/3  "AoA meas (rad)"
  Demux1/2 -> Bus Creator/4  "SS meas (rad)"
  Bus Selector2/4 -> Gain1/1  "<p;q;r>"
  Bus Selector2/5 -> Gain2/1  "<euler>"
  Bus Selector2/6 -> Gain3/1  "<an_b_CG>"
  Gain/1 -> Bus Creator/2  "V_TAS (m/s)"
  Gain1/1 -> Bus Creator/5  "omega_b meas (rad/s)"
  Gain2/1 -> Bus Creator/6  "Euler meas (rad)"
  Gain3/1 -> Bus Creator/7  "an_b_CG meas"
  Bus Creator/1 -> All_measures/1
  Bus Selector2/7 -> Gain4/1  "<Throttle>"
  Gain4/1 -> Bus Creator/8  "Throttle_meas"

== system F16ASYM_Controlled_AoA/Speed-Throttle control ==
  All meas : Inport
  Throttle comm : Inport  Port=2
  delta TAS comm : Inport  Port=3
  "   " : Sum  Inputs=++|
  Add1 : Sum  Inputs=++|
  Manual Switch : ManualSwitch  CurrentSetting=0
  Stall protection TAS : Subsystem
  Throttle Trim Setting : Constant  Value=trim_throttle
  Throttle controller : Subsystem
  V_TAS des : Constant  Value=velocity
  Throttle des : Outport
  TAS des : Outport  Port=2
  wires:
  Throttle controller/1(Throttle des) -> Manual Switch/2
  Add1/1 -> Manual Switch/1
  Throttle Trim Setting/1 -> Add1/1
  Manual Switch/1 -> Throttle des/1
  Stall protection TAS/1(TAS des) -> Throttle controller/1(V_TAS des), TAS des/1
  Throttle comm/1 -> Add1/2
  delta TAS comm/1 -> "   "/2
  V_TAS des/1 -> "   "/1
  "   "/1 -> Stall protection TAS/1(TAS comm)
  All meas/1 -> Stall protection TAS/2(All meas), Throttle controller/2(All meas)

== system F16ASYM_Controlled_AoA/Stall protection A_z and AoA ==
  Reconf param : Inport
  All meas : Inport  Port=2
  A_w_z comm : Inport  Port=3
  AoA comm : Inport  Port=4
  AoA and load factor map : Subsystem  VariantObject=AoA and load factor
  Using AoA : Subsystem  VariantObject=Using AoA
  A_w_z des : Outport
  AoA des : Outport  Port=2

== system F16ASYM_Controlled_AoA/SubSystem3 ==

== system F16ASYM_Controlled_AoA/rad2deg ==
  note: npos,epos,alt
  note: phi
  note: theta
  note: psi
  note: v
  note: alpha
  note: beta
  note: p
  note: q
  note: r
  Params bus : Inport
  States Bus : Inport  Port=2
  Bus Selector : BusSelector  OutputSignals=States_out,Other outs
  Bus Selector1 : BusSelector  OutputSignals=A_w_CG
  Demux1 : Demux  Outputs=[3 1 1 1 1 1 1 1 1 1 1 3 3]
  Gain : Gain  Gain=-1
  Mux : Mux  Inputs=[3 1 1 1 1 1 1 1 1 1 1 3 3 1]
  Mux1 : Mux  Inputs=2
  Selector : Selector  InputPortWidth=3  IndexOptions=Index vector (dialog)  Indices=3  OutputSizes=1
  r2d{,1..7} (8 alike) : Gain  Gain=180/pi  SaturateOnIntegerOverflow=on  OutDataTypeStr=Inherit: Same as input  ParamDataTypeStr=Inherit: Same as input
  Out1 : Outport
  wires:
  Mux1/1 -> Demux1/1
  Demux1/2 -> r2d/1
  Demux1/3 -> r2d1/1
  Demux1/4 -> r2d2/1
  Demux1/1 -> Mux/1
  Demux1/5 -> Mux/5
  r2d2/1 -> Mux/4
  r2d1/1 -> Mux/3
  r2d/1 -> Mux/2
  Demux1/6 -> r2d3/1
  Demux1/7 -> r2d4/1
  Demux1/8 -> r2d5/1
  Demux1/9 -> r2d6/1
  Demux1/10 -> r2d7/1
  r2d4/1 -> Mux/7
  r2d5/1 -> Mux/8
  r2d6/1 -> Mux/9
  r2d7/1 -> Mux/10
  Mux/1 -> Out1/1
  Demux1/12 -> Mux/12  "nx,ny,nz"
  Demux1/13 -> Mux/13  "mach,qbar,ps"
  r2d3/1 -> Mux/6
  Demux1/11 -> Mux/11  "pow"
  Bus Selector/1 -> Mux1/1  "<States_out>"
  Bus Selector/2 -> Mux1/2  "<Other outs>"
  States Bus/1 -> Bus Selector/1
  Params bus/1 -> Bus Selector1/1
  Bus Selector1/1 -> Selector/1  "<A_w_CG>"
  Selector/1 -> Gain/1
  Gain/1 -> Mux/14

== system F16ASYM_Controlled_AoA/Anti-windup Calculation/Anti-windup: NO reconfigurable ==
  note: Reached Angular accel
  note: Converto to Angular accelerations
  Ang accel comm : Inport
  Est reconf : Inport  Port=2
  All_meas : Inport  Port=3
  Surf saturated : Inport  Port=4
  Control_defl : Inport  Port=5
  Analog Filter Design1 : dsparch4/Analog Filter Design  method=Butterworth  filttype=Lowpass  N=8  Wlo=2*pi/T_sim/4  Whi=80  Rp=2  Rs=40
  Analog Filter Design2 : dsparch4/Analog Filter Design  method=Butterworth  filttype=Lowpass  N=8  Wlo=2*pi/T_sim/4  Whi=80  Rp=2  Rs=40
  Analog Filter Design3 : dsparch4/Analog Filter Design  method=Butterworth  filttype=Lowpass  N=8  Wlo=2*pi/T_sim/4  Whi=80  Rp=2  Rs=40
  Ang Accel : MATLAB Function
  Antiwindup calculation : MATLAB Function  TreatAsAtomicUnit=on
  Bus Selector : BusSelector  OutputSignals=signal1.Alt meas (m),signal1.V_TAS (m/s),signal1.AoA meas (rad),signal1.SS meas (rad),signal1.omega_b meas (rad/s),signal1.Throttle_meas
  Bus Selector1 : BusSelector  OutputSignals=signal2.q (Pa),signal1.omega_b meas (rad/s)
  Demux : Demux  Outputs=3
  Demux1 : Demux  Outputs=3
  Effectiveness Matrix B : Constant  Value=B
  Memory1 : Memory  X0=[0,0,0]
  Mom coefficients that was reached : MATLABFcn  MATLABFcn=Moms_Coeff_estimator  OutputDimensions=3  OutputSignalType=real
  Moments : Subsystem
  Mux : Mux  Inputs=3
  Mux1 : Mux  Inputs=7
  Mux2 : Mux  Inputs=3
  Selector : Selector  InputPortWidth=8  IndexOptions=Index vector (dialog)  Indices=1:7  OutputSizes=1
  Terminator1 : Terminator
  Anti-windup signals : Outport
  wires:
  Selector/1 -> Antiwindup calculation/5(deflections), Mux1/7
  Mux1/1 -> Mom coefficients that was reached/1
  Bus Selector/5 -> Mux1/5  "<omega_b meas (rad/s)>"
  Bus Selector/1 -> Mux1/1  "<Alt meas (m)>"
  Bus Selector/2 -> Mux1/2  "<V_TAS (m/s)>"
  Bus Selector/3 -> Mux1/3  "<AoA meas (rad)>"
  Bus Selector/4 -> Mux1/4  "<SS meas (rad)>"
  Control_defl/1 -> Selector/1
  Bus Selector/6 -> Mux1/6  "<Throttle_meas>"
  Ang Accel/2(q_dot) -> Mux/2
  Ang Accel/3(r_dot) -> Mux/3
  Ang Accel/1(p_dot) -> Mux/1
  Bus Selector1/2 -> Ang Accel/4(omega_b)  "<omega_b meas (rad/s)>"
  Moments/3(N) -> Ang Accel/3(N)
  Moments/2(M) -> Ang Accel/2(M)
  Moments/1(L) -> Ang Accel/1(L)
  Bus Selector1/1 -> Moments/4(q)  "<q (Pa)>"
  Demux/3 -> Moments/3(C_N)
  Demux/2 -> Moments/2(C_M)
  Demux/1 -> Moments/1(C_L)
  Mom coefficients that was reached/1 -> Demux/1
  All_meas/1 -> Bus Selector/1, Bus Selector1/1
  Est reconf/1 -> Terminator1/1
  Mux/1 -> Antiwindup calculation/2(Ang_acell_achieved)
  Effectiveness Matrix B/1 -> Antiwindup calculation/4(B)
  Surf saturated/1 -> Antiwindup calculation/3(Saturations)
  Ang accel comm/1 -> Memory1/1
  Memory1/1 -> Antiwindup calculation/1(Ang_acell_comm)
  Mux2/1 -> Anti-windup signals/1
  Antiwindup calculation/1(AWU) -> Demux1/1
  Demux1/1 -> Analog Filter Design3/1
  Demux1/2 -> Analog Filter Design1/1
  Analog Filter Design3/1 -> Mux2/1
  Analog Filter Design1/1 -> Mux2/2
  Analog Filter Design2/1 -> Mux2/3
  Demux1/3 -> Analog Filter Design2/1
